simulink model "SS_F16_Block"  (Simulink 5.0)
settings: Solver=ode5  StartTime=0.0  StopTime=30.0  FixedStep=deltaT  RelTol=1e-3
undefined symbols (not defined in the file): A, B, C, D, DisAil_1, DisAil_2, DisAil_3, DisEle_1, DisEle_2, DisEle_3, DisRud_1, DisRud_2, DisRud_3, thrust, trim_control, trim_state, trim_thrust
settings Model: Creator=russ1110  LastModifiedBy=rrussell  ExtModeAutoUpdateStatusClock=off  BooleanDataType=off

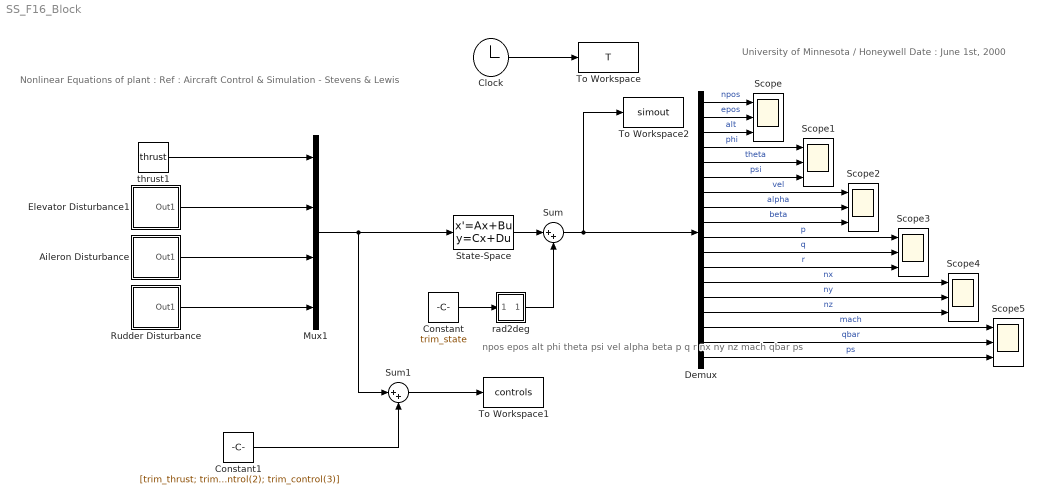
== system SS_F16_Block ==
  note: npos
      | epos
      | alt
      | phi
      | theta
      | psi
      | vel
      | alpha
      | beta
      | p
      | q
      | r
      | nx
      | ny
      | nz
      | mach
      | qbar
      | ps
  note: University of Minnesota / Honeywell
      | Date : June 1st, 2000
  note: Nonlinear Equations of plant :
      | Ref : Aircraft Control & Simulation
      | - Stevens & Lewis
  Aileron Disturbance : Subsystem
  Clock : Clock
      settings: Decimation=50
  Constant : Constant  Value=trim_state
  Constant1 : Constant  Value=[trim_thrust; trim_control(1); trim_control(2); trim_control(3)]
  Demux : Demux  Outputs=18
  Elevator Disturbance1 : Subsystem
  Mux1 : Mux
  Rudder Disturbance : Subsystem
  Scope{,1..5} (6 alike) : Scope  NumInputPorts=3
      Scope settings: YMin=-5~-5~-5  YMax=5~5~5  Decimation=20
      Scope1 settings: YMin=-5~-5~-5  YMax=5~5~5  Decimation=20
      Scope2 settings: YMin=-5~-5~-5  YMax=5~5~5  SaveName=ScopeData2  Decimation=20
      Scope3 settings: YMin=-5~-5~-5  YMax=5~5~5  SaveName=ScopeData3  Decimation=20
      Scope4 settings: YMin=-5~-5~-5  YMax=5~5~5  SaveName=ScopeData4  Decimation=20
      Scope5 settings: YMin=-5~-5~-5  YMax=5~5~5  SaveName=ScopeData5
  State-Space : StateSpace  A=A  B=B  C=C  D=D
  Sum : Sum  Inputs=|++  SaturateOnIntegerOverflow=on  InputSameDT=on
  Sum1 : Sum  Inputs=|++  SaturateOnIntegerOverflow=on  InputSameDT=on
  To Workspace : ToWorkspace  VariableName=T  SampleTime=-1  SaveFormat=Array
      settings: Decimation=100
  To Workspace1 : ToWorkspace  VariableName=controls  SampleTime=-1  SaveFormat=Array
      settings: Decimation=100
  To Workspace2 : ToWorkspace  VariableName=simout  SampleTime=-1  SaveFormat=Array
      settings: Decimation=100
  rad2deg : Subsystem
  thrust1 : Constant  Value=thrust  VectorParams1D=off
  wires:
  Clock/1 -> To Workspace/1
  Demux/1 -> Scope/1  "npos"
  Demux/2 -> Scope/2  "epos"
  Demux/3 -> Scope/3  "alt"
  Demux/5 -> Scope1/2  "theta"
  Demux/6 -> Scope1/3  "psi"
  Demux/7 -> Scope2/1  "vel"
  Demux/8 -> Scope2/2  "alpha"
  Demux/9 -> Scope2/3  "beta"
  Demux/10 -> Scope3/1  "p"
  Demux/11 -> Scope3/2  "q"
  Demux/12 -> Scope3/3  "r"
  Demux/13 -> Scope4/1  "nx"
  Demux/14 -> Scope4/2  "ny"
  Demux/15 -> Scope4/3  "nz"
  Demux/4 -> Scope1/1  "phi"
  Demux/16 -> Scope5/1  "mach"
  Demux/17 -> Scope5/2  "qbar"
  Demux/18 -> Scope5/3  "ps"
  State-Space/1 -> Sum/1
  Sum/1 -> Demux/1, To Workspace2/1
  thrust1/1 -> Mux1/1
  Elevator Disturbance1/1(Out1) -> Mux1/2
  Aileron Disturbance/1(Out1) -> Mux1/3
  Rudder Disturbance/1(Out1) -> Mux1/4
  Constant1/1 -> Sum1/2
  Mux1/1 -> State-Space/1, Sum1/1
  Sum1/1 -> To Workspace1/1
  rad2deg/1(Out1) -> Sum/2
  Constant/1 -> rad2deg/1(In1)

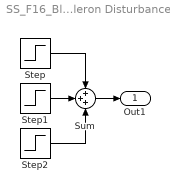
== system SS_F16_Block/Aileron Disturbance ==
  Step : Step  After=DisAil_1  SampleTime=0
  Step1 : Step  Time=3  After=DisAil_2  SampleTime=0
  Step2 : Step  Time=5  After=DisAil_3  SampleTime=0
  Sum : Sum  Inputs=+++  SaturateOnIntegerOverflow=on  InputSameDT=on
  Out1 : Outport
  wires:
  Step1/1 -> Sum/2
  Step/1 -> Sum/1
  Step2/1 -> Sum/3
  Sum/1 -> Out1/1

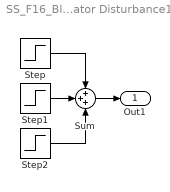
== system SS_F16_Block/Elevator Disturbance1 ==
  Step : Step  After=DisEle_1  SampleTime=0
  Step1 : Step  Time=3  After=DisEle_2  SampleTime=0
  Step2 : Step  Time=5  After=DisEle_3  SampleTime=0
  Sum : Sum  Inputs=+++  SaturateOnIntegerOverflow=on  InputSameDT=on
  Out1 : Outport
  wires:
  Step1/1 -> Sum/2
  Step/1 -> Sum/1
  Step2/1 -> Sum/3
  Sum/1 -> Out1/1

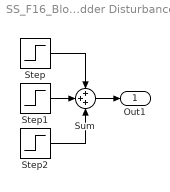
== system SS_F16_Block/Rudder Disturbance ==
  Step : Step  After=DisRud_1  SampleTime=0
  Step1 : Step  Time=1.5  After=DisRud_2  SampleTime=0
  Step2 : Step  Time=2  After=DisRud_3  SampleTime=0
  Sum : Sum  Inputs=+++  SaturateOnIntegerOverflow=on  InputSameDT=on
  Out1 : Outport
  wires:
  Step1/1 -> Sum/2
  Step/1 -> Sum/1
  Step2/1 -> Sum/3
  Sum/1 -> Out1/1

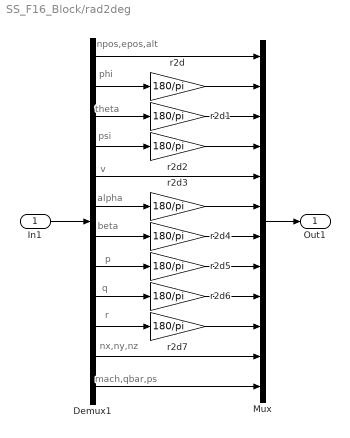
== system SS_F16_Block/rad2deg ==
  note: npos,epos,alt
  note: phi
  note: theta
  note: psi
  note: v
  note: alpha
  note: beta
  note: p
  note: q
  note: r
  note: nx,ny,nz
  note: mach,qbar,ps
  In1 : Inport
  Demux1 : Demux  Outputs=[3 1 1 1 1 1 1 1 1 1 3 3]
  Mux : Mux  Inputs=[3 1 1 1 1 1 1 1 1 1 3 3]
  r2d{,1..7} (8 alike) : Gain  Gain=180/pi  SaturateOnIntegerOverflow=on
  Out1 : Outport
  wires:
  In1/1 -> Demux1/1
  Demux1/2 -> r2d/1
  Demux1/3 -> r2d1/1
  Demux1/4 -> r2d2/1
  Demux1/1 -> Mux/1
  Demux1/5 -> Mux/5
  r2d2/1 -> Mux/4
  r2d1/1 -> Mux/3
  r2d/1 -> Mux/2
  Demux1/6 -> r2d3/1
  Demux1/7 -> r2d4/1
  Demux1/8 -> r2d5/1
  Demux1/9 -> r2d6/1
  Demux1/10 -> r2d7/1
  r2d3/1 -> Mux/6
  r2d4/1 -> Mux/7
  r2d5/1 -> Mux/8
  r2d6/1 -> Mux/9
  r2d7/1 -> Mux/10
  Mux/1 -> Out1/1
  Demux1/11 -> Mux/11
  Demux1/12 -> Mux/12
